simulink model "Problem_5"  (R2020a)
settings: Solver=VariableStepAuto  StartTime=0.0  StopTime=10.0  RelTol=1e-3
model workspace (MAT data in the model file):
  C1 = 1e-06
  R1 = 10
settings Model: Creator=user  LastModifiedBy=user

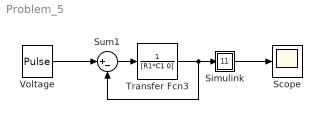
== system Problem_5 ==
  Scope : Scope
  Simulink : Subsystem
      mask Display: disp('V')
  Sum1 : Sum  Inputs=|+-
  Transfer Fcn3 : TransferFcn  InitFcn=wp=1/(R*C);  Denominator=[R1*C1 0]
  Voltage : DiscretePulseGenerator  PulseType=Time based  Amplitude=2  Period=3  PulseWidth=50  PhaseDelay=1e-3
  wires:
  Sum1/1 -> Transfer Fcn3/1
  Transfer Fcn3/1 -> Simulink/1(In1), Sum1/2
  Voltage/1 -> Sum1/1
  Simulink/1(Out) -> Scope/1

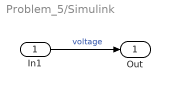
== system Problem_5/Simulink ==
  In1 : Inport
  Out : Outport  VectorParamsAs1DForOutWhenUnconnected=off
  wires:
  In1/1 -> Out/1  "voltage"
